simulink model "PIDModel"  (R2021a)
settings: Solver=VariableStepAuto  StartTime=0.0  StopTime=20  FixedStep=0.02  RelTol=1e-3
model workspace (MAT data in the model file):
  D = 0.711
  DragCoeff = 4e-05
  J = 0.003408
  Ke = 0.0796
  Kt = 0.079
  La = 4.55e-05
  LiftCoeff = 0.0026
  Ra = 0.06
  Rho = 1.2256
  kf = 0.03408
libraries: pid_lib x1
settings Model: Creator=js20164  LastModifiedBy=james
settings SolverCC: AlgebraicLoopSolver=TrustRegion
settings DebuggingCC: SFMachineParentedDataDiag=warning

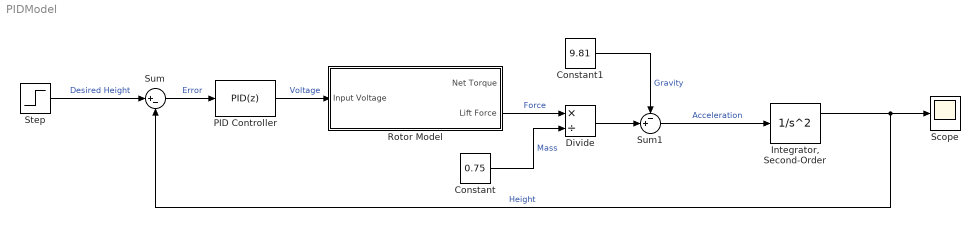
== system PIDModel ==
  Constant : Constant  Value=0.75
  Constant1 : Constant  Value=9.81
  Divide : Product  Inputs=*/
  "Integrator, Second-Order" : SecondOrderIntegrator
  PID Controller : pid_lib/PID Controller  Controller=PID  Form=Parallel  TimeDomain=Discrete-time  UseExternalTs=off  SampleTime=0.02  IntegratorMethod=Forward Euler  FilterMethod=Forward Euler  ControllerParametersSource=internal  P=4  I=3  D=1  UseFilter=off  N=1  TunerSelectOption=Frequency Response Based  InitialConditionSource=internal  InitialConditionForIntegrator=0  InitialConditionForFilter=0  DifferentiatorICPrevScaledInput=0  ExternalReset=none  TrackingMode=off  Kt=1  LimitOutput=on  SatLimitsSource=internal  UpperSaturationLimit=44.4  LowerSaturationLimit=0  LinearizeAsGain=on  AntiWindupMode=clamping  Kb=1  POutMin=[]  POutMax=[]  IOutMin=[]  IOutMax=[]  DOutMin=[]  DOutMax=[]  NOutMin=[]  NOutMax=[]  SumOutMin=[]  SumOutMax=[]  SaturationOutMin=[]  SaturationOutMax=[]  PParamMin=[]  PParamMax=[]  IParamMin=[]  IParamMax=[]  DParamMin=[]  DParamMax=[]  NParamMin=[]  NParamMax=[]  KbParamMin=[]  KbParamMax=[]  KtParamMin=[]  KtParamMax=[]  KbOutMin=[]  KbOutMax=[]  KtOutMin=[]  KtOutMax=[]  IntegratorOutMin=[]  IntegratorOutMax=[]  FilterOutMin=[]  FilterOutMax=[]  SumI1OutMin=[]  SumI1OutMax=[]  SumI2OutMin=[]  SumI2OutMax=[]  SumI3OutMin=[]  SumI3OutMax=[]  SumI4OutMin=[]  SumI4OutMax=[]  SumDOutMin=[]  SumDOutMax=[]  DifferentiatorOutMin=[]  DifferentiatorOutMax=[]  FilterDiffOutCoefMin=[]  FilterDiffOutCoefMax=[]  ReciprocalOutMin=[]  ReciprocalOutMax=[]  SumDenOutMin=[]  SumDenOutMax=[]  SumNumOutMin=[]  SumNumOutMax=[]  DivideOutMin=[]  DivideOutMax=[]  UdiffTsProdOutMin=[]  UdiffTsProdOutMax=[]  NTsProdOutMin=[]  NTsProdOutMax=[]  UintegralTsProdOutMin=[]  UintegralTsProdOutMax=[]  UngainTsProdOutMin=[]  UngainTsProdOutMax=[]  IntegratorContinuousStateAttributes=''  IntegratorStateMustResolveToSignalObject=off  IntegratorRTWStateStorageClass=Auto  FilterContinuousStateAttributes=''  FilterStateMustResolveToSignalObject=off  FilterRTWStateStorageClass=Auto  ParallelPVariant=InternalParameters  IdealPVariant=Disabled  IVariant=InternalParameters  DVariant=InternalParameters  IntegratorVariant=Discrete  SatVariant=Enabled  AWVariant=DiscClampingParallel  PCopyVariant=Disabled  TRVariant=Disabled  FdbkBlocksVariant=Forward  IdealPFdbkVariant=Disabled  SatFdbkVariant=Disabled  DerivativeFilterVariant=Differentiator  NVariant=Passthrough  NCopyVariant=Disabled_SignalSpec  FilterICVariant=InternalICsDifferentiator  IntegratorICVariant=InternalICs  ExternalResetVariant=Disabled  TRSumVariant=Passthrough  SumFdbkVariant=Disabled  SumVariant=Sum_PID  TsampFilterVariant=InternalTs  TsampNgainVariant=Passthrough  TsampIntegralVariant=Passthrough  ExternalSaturationOutDataTypeStr=Inherit: Same as second input
  Rotor Model : Subsystem
  Scope : Scope
  Step : Step  Time=0.1  After=30  SampleTime=0
  Sum : Sum  Inputs=|+-
  Sum1 : Sum  Inputs=-+|
  wires:
  Rotor Model/2(Lift Force) -> Divide/1  "Force"
  Constant/1 -> Divide/2  "Mass"
  "Integrator, Second-Order"/1 -> Sum/2, Scope/1  "Height"
  Step/1 -> Sum/1  "Desired Height"
  Divide/1 -> Sum1/2
  Sum1/1 -> "Integrator, Second-Order"/1  "Acceleration"
  Constant1/1 -> Sum1/1  "Gravity"
  Sum/1 -> PID Controller/1  "Error"
  PID Controller/1 -> Rotor Model/1(Input Voltage)  "Voltage"

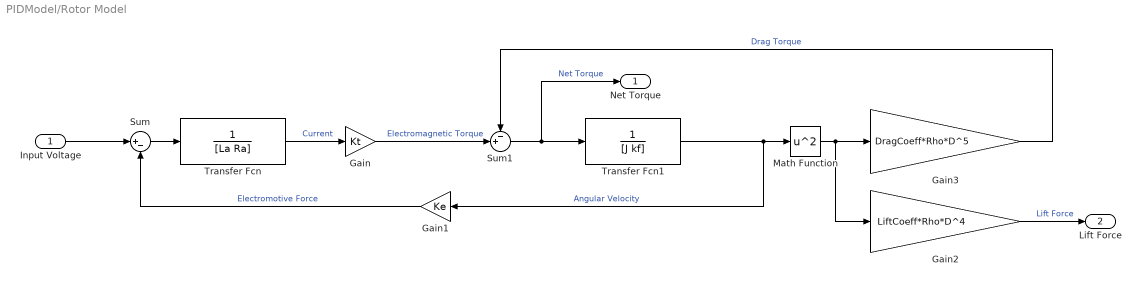
== system PIDModel/Rotor Model ==
  Input Voltage : Inport
  Gain : Gain  Gain=Kt
  Gain1 : Gain  Gain=Ke
  Gain2 : Gain  Gain=LiftCoeff*Rho*D^4
  Gain3 : Gain  Gain=DragCoeff*Rho*D^5
  Math Function : Math  Operator=square  SaturateOnIntegerOverflow=on
  Sum : Sum  Inputs=|+-
  Sum1 : Sum  Inputs=-+|
  Transfer Fcn : TransferFcn  Denominator=[La Ra]
  Transfer Fcn1 : TransferFcn  Denominator=[J kf]
  Net Torque : Outport
  Lift Force : Outport  Port=2
  wires:
  Gain1/1 -> Sum/2  "Electromotive Force"
  Sum/1 -> Transfer Fcn/1
  Gain2/1 -> Lift Force/1  "Lift Force"
  Gain3/1 -> Sum1/1  "Drag Torque"
  Gain/1 -> Sum1/2  "Electromagnetic Torque"
  Sum1/1 -> Net Torque/1, Transfer Fcn1/1  "Net Torque"
  Transfer Fcn1/1 -> Gain1/1, Math Function/1  "Angular Velocity"
  Math Function/1 -> Gain3/1, Gain2/1
  Transfer Fcn/1 -> Gain/1  "Current"
  Input Voltage/1 -> Sum/1
